simulink model "bd_btyrc"  (Simulink 3.00)
settings: Solver=ode1  SolverMode=SingleTasking  StartTime=0.0  StopTime=100000  FixedStep=1  MaxStep=1  RelTol=1e-3  AbsTol=1e-3
values from neighbouring files (symbols this model uses):
  amb_tmp = vinf.test.ambtmp    [RW_execute.m]
  ess_init_soc = vinf.test.ess_init_soc.FUDS    [J17_FUDS.m]    (also in J17_HFEDS.m = vinf.test.ess_init_soc.HWFET; J17_SC03.m = vinf.test.ess_init_soc.SC03; J17_UDDS.m = vinf.test.ess_init_soc.UDDS; J17_US06.m = vinf.test.ess_init_soc.US06)
undefined symbols (not defined in the file or in its folder): ess_coulombic_eff, ess_max_ah_cap, ess_module_num, ess_tmp
CloseFcn:
  | ;slview('closediagram',bdroot);
settings Model: SaveTime=off  SaveOutput=off  LastModifiedBy=tmarkel

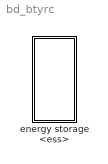
== system bd_btyrc ==
  energy storage <ess> : Subsystem

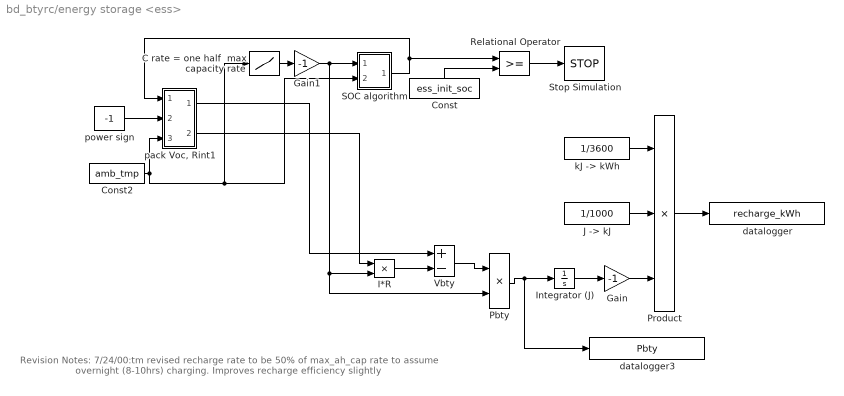
== system bd_btyrc/energy storage <ess> ==
  note: Revision Notes:
      | 7/24/00:tm revised recharge rate to be 50% of max_ah_cap
      | rate to assume overnight (8-10hrs) charging.
      | Improves recharge efficiency slightly
  C rate = one half  max capacity rate : Lookup  InputValues=ess_tmp  OutputValues=ess_max_ah_cap/2
  Const : Constant  Orientation=up  Value=ess_init_soc
  Const2 : Constant  Value=amb_tmp
  Gain : Gain  Gain=-1  SaturateOnIntegerOverflow=on
  Gain1 : Gain  Gain=-1  SaturateOnIntegerOverflow=on
  I*R : Product  Inputs=2  SaturateOnIntegerOverflow=on
  Integrator (J) : Integrator  ExternalReset=none  InitialConditionSource=internal  InitialCondition=0  LimitOutput=off  UpperSaturationLimit=inf  LowerSaturationLimit=-inf  ShowSaturationPort=off  ShowStatePort=off  AbsoluteTolerance=auto
  "J -> kJ" : Constant  Value=1/1000
  Pbty : Product  Inputs=2  SaturateOnIntegerOverflow=on
  Product : Product  Inputs=3  SaturateOnIntegerOverflow=on
  Relational Operator : RelationalOperator  Operator=>=
  SOC algorithm : Subsystem
  Stop Simulation : Stop
  Vbty : Sum  Inputs=+-  SaturateOnIntegerOverflow=on
  datalogger : ToWorkspace  VariableName=recharge_kWh  SampleTime=0  SaveFormat=Matrix
      settings: Buffer=1
  datalogger3 : ToWorkspace  VariableName=Pbty  SampleTime=0  SaveFormat=Matrix
      settings: Buffer=1
  "kJ -> kWh" : Constant  Value=1/3600
  "pack Voc, Rint1" : Subsystem
  power sign : Constant  Value=-1
  wires:
  power sign/1 -> "pack Voc, Rint1"/2(req'd battery power (W))
  Relational Operator/1 -> Stop Simulation/1
  Const/1 -> Relational Operator/2
  I*R/1 -> Vbty/2
  Vbty/1 -> Pbty/1
  "kJ -> kWh"/1 -> Product/1
  Product/1 -> datalogger/1
  Integrator (J)/1 -> Gain/1
  Pbty/1 -> Integrator (J)/1, datalogger3/1
  "J -> kJ"/1 -> Product/2
  Gain/1 -> Product/3
  "pack Voc, Rint1"/1(pack open- circuit voltage) -> Vbty/1
  "pack Voc, Rint1"/2(pack resistance) -> I*R/1
  SOC algorithm/1(SOC1) -> "pack Voc, Rint1"/1(SOC (prev)), Relational Operator/1
  Const2/1 -> "pack Voc, Rint1"/3(mod tmp   (C)), SOC algorithm/2(tmp (C)), C rate = one half  max capacity rate/1
  C rate = one half  max capacity rate/1 -> Gain1/1
  Gain1/1 -> SOC algorithm/1((A)), I*R/2, Pbty/2

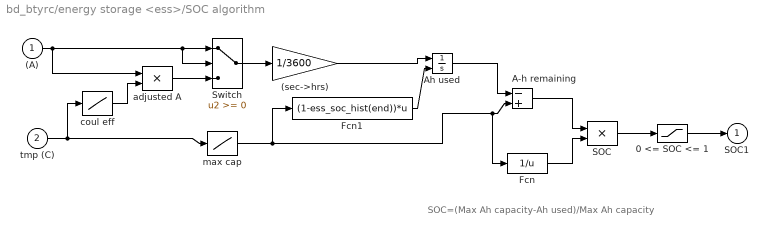
== system bd_btyrc/energy storage <ess>/SOC algorithm ==
  note: SOC=(Max Ah capacity-Ah used)/Max Ah capacity
  (A) : Inport  Port=1  PortWidth=-1  SampleTime=-1  DataType=auto
      settings: SignalType=auto
  tmp (C) : Inport  Port=2  PortWidth=-1  SampleTime=-1  DataType=auto
      settings: SignalType=auto
  (sec->hrs) : Gain  Gain=1/3600  SaturateOnIntegerOverflow=on
  0 <= SOC <= 1 : Saturate  UpperLimit=1  LowerLimit=0
  A-h remaining : Sum  Inputs=-+  SaturateOnIntegerOverflow=on
  Ah used : Integrator  ExternalReset=none  InitialConditionSource=external  InitialCondition=(1-ess_init_soc)*ess_max_ah_cap  LimitOutput=off  UpperSaturationLimit=inf  LowerSaturationLimit=-inf  ShowSaturationPort=off  ShowStatePort=off  AbsoluteTolerance=auto
  Fcn : Fcn  Expr=1/u
  Fcn1 : Fcn  Expr=(1-ess_soc_hist(end))*u
  SOC : Product  Inputs=2  SaturateOnIntegerOverflow=on
  Switch : Switch  Threshold=0
  adjusted A : Product  Inputs=2  SaturateOnIntegerOverflow=on
  coul eff : Lookup  InputValues=ess_tmp  OutputValues=ess_coulombic_eff
  max cap : Lookup  InputValues=ess_tmp  OutputValues=ess_max_ah_cap
  SOC1 : Outport  Port=1  InitialOutput=0
  wires:
  (A)/1 -> Switch/2, Switch/1, adjusted A/1
  Switch/1 -> (sec->hrs)/1
  (sec->hrs)/1 -> Ah used/1
  Ah used/1 -> A-h remaining/1
  Fcn/1 -> SOC/2
  SOC/1 -> 0 <= SOC <= 1/1
  A-h remaining/1 -> SOC/1
  0 <= SOC <= 1/1 -> SOC1/1
  tmp (C)/1 -> max cap/1, coul eff/1
  coul eff/1 -> adjusted A/2
  adjusted A/1 -> Switch/3
  max cap/1 -> A-h remaining/2, Fcn/1, Fcn1/1
  Fcn1/1 -> Ah used/2

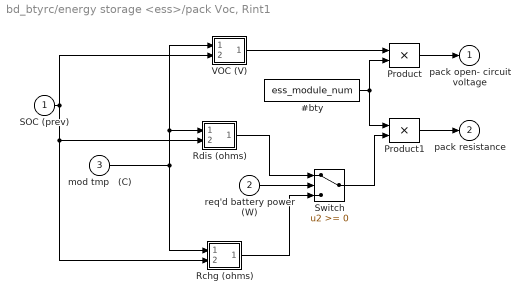
== system bd_btyrc/energy storage <ess>/pack Voc, Rint1 ==
  SOC (prev) : Inport  Port=1  PortWidth=-1  SampleTime=-1  DataType=auto
      settings: SignalType=auto
  req'd battery power (W) : Inport  Port=2  PortWidth=-1  SampleTime=-1  DataType=auto
      settings: SignalType=auto
  mod tmp   (C) : Inport  Port=3  PortWidth=-1  SampleTime=-1  DataType=auto
      settings: SignalType=auto
  #bty : Constant  Value=ess_module_num
  Product : Product  Inputs=2  SaturateOnIntegerOverflow=on
  Product1 : Product  Inputs=2  SaturateOnIntegerOverflow=on
  Rchg (ohms) : Subsystem  mask(2-D Table Lookup){@1=ess_tmp, @2=ess_soc, @3=ess_r_chg}
      mask prompts: @1 "X Index"; @2 "Y Index"; @3 "Table"
      mask help:
      | Two Dimensional Table Lookup
      | The first input corresponds to X Index and the second input corresponds to the Y Index
      mask init:
      | xindex=@1; yindex=@2; table=@3; sftab2chk(xindex,yindex,table);
      mask Help: This block returns a linearly interpolated intersection from the table using the X index (which corresponds to the rows of the table) and the Y index (which corresponds to the columns of the table).  Extrapolation is used.
      mask Display: plot(-10,-10,110,110,[90,50,10],[90,40,30],[90,50,10],[50,26,20],[90,50,10],[22,13,10])
  Rdis (ohms) : Subsystem  mask(2-D Table Lookup){@1=ess_tmp, @2=ess_soc, @3=ess_r_dis}
      mask prompts: @1 "X Index"; @2 "Y Index"; @3 "Table"
      mask help:
      | Two Dimensional Table Lookup
      | The first input corresponds to X Index and the second input corresponds to the Y Index
      mask init:
      | xindex=@1; yindex=@2; table=@3; sftab2chk(xindex,yindex,table);
      mask Help: This block returns a linearly interpolated intersection from the table using the X index (which corresponds to the rows of the table) and the Y index (which corresponds to the columns of the table).  Extrapolation is used.
      mask Display: plot(-10,-10,110,110,[90,50,10],[90,40,30],[90,50,10],[50,26,20],[90,50,10],[22,13,10])
  Switch : Switch  Threshold=0
  VOC (V) : Subsystem  mask(2-D Table Lookup){@1=ess_tmp, @2=ess_soc, @3=ess_voc}
      mask prompts: @1 "X Index"; @2 "Y Index"; @3 "Table"
      mask help:
      | Two Dimensional Table Lookup
      | The first input corresponds to X Index and the second input corresponds to the Y Index
      mask init:
      | xindex=@1; yindex=@2; table=@3; sftab2chk(xindex,yindex,table);
      mask Help: This block returns a linearly interpolated intersection from the table using the X index (which corresponds to the rows of the table) and the Y index (which corresponds to the columns of the table).  Extrapolation is used.
      mask Display: plot(-10,-10,110,110,[90,50,10],[90,40,30],[90,50,10],[50,26,20],[90,50,10],[22,13,10])
  pack open- circuit voltage : Outport  Port=1  InitialOutput=0
  pack resistance : Outport  Port=2  InitialOutput=0
  wires:
  Product/1 -> pack open- circuit voltage/1
  Product1/1 -> pack resistance/1
  #bty/1 -> Product1/1, Product/2
  VOC (V)/1(table out) -> Product/1
  Rchg (ohms)/1(table out) -> Switch/3
  Rdis (ohms)/1(table out) -> Switch/1
  req'd battery power (W)/1 -> Switch/2
  Switch/1 -> Product1/2
  SOC (prev)/1 -> VOC (V)/2(y0), Rdis (ohms)/2(y0), Rchg (ohms)/2(y0)
  mod tmp   (C)/1 -> VOC (V)/1(x0), Rdis (ohms)/1(x0), Rchg (ohms)/1(x0)

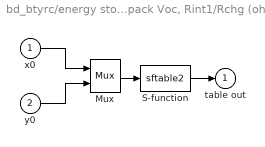
== system bd_btyrc/energy storage <ess>/pack Voc, Rint1/Rchg (ohms) ==
  x0 : Inport  Port=1  PortWidth=-1  SampleTime=-1  DataType=auto
      settings: SignalType=auto
  y0 : Inport  Port=2  PortWidth=-1  SampleTime=-1  DataType=auto
      settings: SignalType=auto
  Mux : Mux  Inputs=2
      settings: DisplayOption=none
  S-function : S-Function  FunctionName=sftable2  Parameters=xindex, yindex, table  PortCounts=[]  SFunctionModules=''
  table out : Outport  Port=1  InitialOutput=0
  wires:
  y0/1 -> Mux/2
  S-function/1 -> table out/1
  x0/1 -> Mux/1
  Mux/1 -> S-function/1

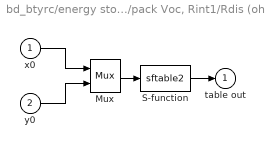
== system bd_btyrc/energy storage <ess>/pack Voc, Rint1/Rdis (ohms) ==
  x0 : Inport  Port=1  PortWidth=-1  SampleTime=-1  DataType=auto
      settings: SignalType=auto
  y0 : Inport  Port=2  PortWidth=-1  SampleTime=-1  DataType=auto
      settings: SignalType=auto
  Mux : Mux  Inputs=2
      settings: DisplayOption=none
  S-function : S-Function  FunctionName=sftable2  Parameters=xindex, yindex, table  PortCounts=[]  SFunctionModules=''
  table out : Outport  Port=1  InitialOutput=0
  wires:
  y0/1 -> Mux/2
  S-function/1 -> table out/1
  x0/1 -> Mux/1
  Mux/1 -> S-function/1

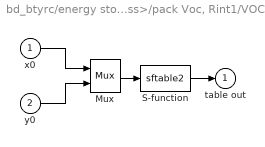
== system bd_btyrc/energy storage <ess>/pack Voc, Rint1/VOC (V) ==
  x0 : Inport  Port=1  PortWidth=-1  SampleTime=-1  DataType=auto
      settings: SignalType=auto
  y0 : Inport  Port=2  PortWidth=-1  SampleTime=-1  DataType=auto
      settings: SignalType=auto
  Mux : Mux  Inputs=2
      settings: DisplayOption=none
  S-function : S-Function  FunctionName=sftable2  Parameters=xindex, yindex, table  PortCounts=[]  SFunctionModules=''
  table out : Outport  Port=1  InitialOutput=0
  wires:
  y0/1 -> Mux/2
  S-function/1 -> table out/1
  x0/1 -> Mux/1
  Mux/1 -> S-function/1
